simulink model "real"  (R2023a)
settings: Solver=ode1  StartTime=0.0  StopTime=inf  FixedStep=0.005  RelTol=1e-3
settings Model: SimulationMode=external  ExtModeTrigDuration=200000  Creator=5420  LastModifiedBy=zhs20
settings SolverCC: AlgebraicLoopSolver=TrustRegion
settings DataIOCC: LimitDataPoints=on  SaveFormat=Array  SignalLoggingSaveFormat=ModelDataLogs  ReturnWorkspaceOutputs=off  SignalLoggingName=sigsOut
settings OptimizationCC: ExpressionDepthLimit=2147483647  InitFltsAndDblsToZero=on
settings DebuggingCC: SaveWithParameterizedLinksMsg=none  UnderspecifiedInitializationDetection=Classic  MergeDetectMultiDrivingBlocksExec=none  SignalResolutionControl=TryResolveAllWithWarning  MultiTaskDSMMsg=warning  MultiTaskCondExecSysMsg=none  UnconnectedInputMsg=warning  UnconnectedOutputMsg=warning  UnconnectedLineMsg=warning  StateNameClashWarn=warning  SFUnexpectedBacktrackingDiag=warning  SFNoUnconditionalDefaultTransitionDiag=warning  SFExecutionAtInitializationDiag=none  ArithmeticOperatorsInVariantConditions=warning
settings HardwareCC: ProdBitPerLong=64  ProdHWDeviceType=Intel->x86-64 (Linux 64)
settings ModelReferenceCC: PropagateSignalLabelsOutOfModel=off
settings SFSimCC: SimUseLocalCustomCode=off  CustomCodeUndefinedFunction=UseInterfaceOnly
settings RTWCC: Description=Simulink Desktop Real-Time  SystemTargetFile=sldrt.tlc  TemplateMakefile=sldrt.tmf  RTWUseLocalCustomCode=off  RTWCompilerOptimization=on
settings CodeAppCC: MaxIdLength=95  StateflowObjectComments=on
settings SimulinkDesktopRealTimeCC: TargetLibSuffix=_sldrt.a  TargetPreCompLibLocation=C:\Program Files\MATLAB\R2023a\toolbox\sldrt\lib\win64  TargetLangStandard=C89/C90 (ANSI)  ModelReferenceCompliant=off  CompOptLevelCompliant=off  SupportVariableSizeSignals=off
settings ConfigComp: CovMetricSettings=dw  CovSaveCumulativeToWorkspaceVar=on  CovSaveSingleToWorkspaceVar=on  CovExternalEMLEnable=off

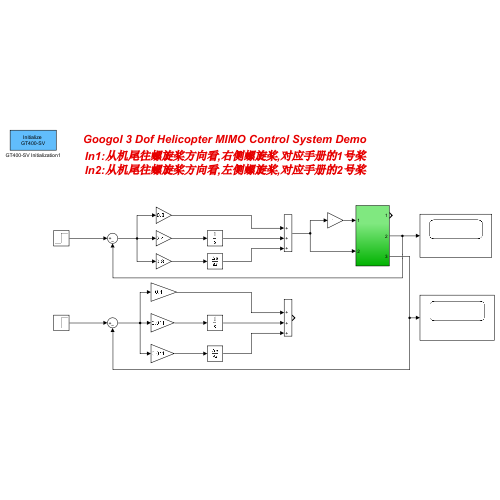
[thumbnail: Simulink's stored preview of the top-level diagram]
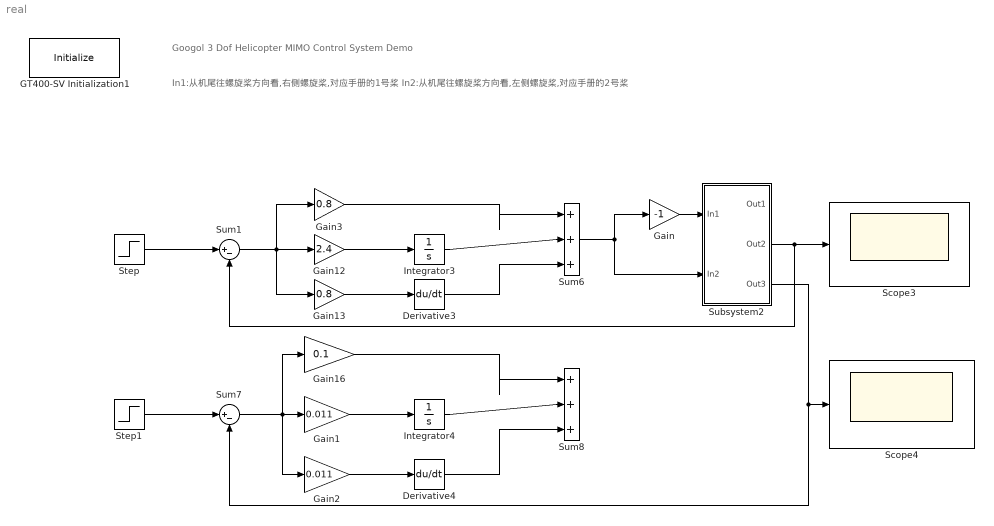
== system real ==
  note: Googol 3 Dof Helicopter MIMO Control System Demo
  note: In1:从机尾往螺旋桨方向看,右侧螺旋桨,对应手册的1号桨
      | In2:从机尾往螺旋桨方向看,左侧螺旋桨,对应手册的2号桨
  Derivative3 : Derivative
  Derivative4 : Derivative
  GT400-SV Initialization1 : S-Function  Priority=0  FunctionName=Initialize  Parameters=openloop  SFunctionDeploymentMode=off  EnableBusSupport=off  mask(Initialize){openloop=1}
      mask prompts: openloop "Control loop:"
      mask help:
      | Initializing the googol GT400-SV motion control board.
      | Block parameter:
      |     Control loop:
      |          0: closed-loop control.
      |          1: opened-loop control.
      mask Help: This initialize block initializes the googol GT400-SV motion control board.
      mask Display: disp('Initialize \nGT400-SV');
  Gain : Gain  Gain=-1
  Gain1 : Gain  Gain=0.011
  Gain12 : Gain  Gain=2.4
  Gain13 : Gain  Gain=0.8
  Gain16 : Gain  Gain=0.1
  Gain2 : Gain  Gain=0.011
  Gain3 : Gain  Gain=0.8
  Integrator3 : Integrator
  Integrator4 : Integrator
  Scope3 : Scope
  Scope4 : Scope
  Step : Step  After=0.3  SampleTime=0
  Step1 : Step  After=3  SampleTime=0
  Subsystem2 : Subsystem
  Sum1 : Sum  Inputs=|+-
  Sum6 : Sum  Inputs=|+++
  Sum7 : Sum  Inputs=|+-
  Sum8 : Sum  Inputs=|+++
  wires:
  Sum1/1 -> Gain3/1, Gain12/1, Gain13/1
  Gain12/1 -> Integrator3/1
  Gain13/1 -> Derivative3/1
  Gain3/1 -> Sum6/1
  Integrator3/1 -> Sum6/2
  Derivative3/1 -> Sum6/3
  Subsystem2/2(Out2) -> Scope3/1, Sum1/2
  Step1/1 -> Sum7/1
  Sum7/1 -> Gain2/1, Gain1/1, Gain16/1
  Gain1/1 -> Integrator4/1
  Gain2/1 -> Derivative4/1
  Gain16/1 -> Sum8/1
  Integrator4/1 -> Sum8/2
  Derivative4/1 -> Sum8/3
  Sum6/1 -> Gain/1, Subsystem2/2(In2)
  Gain/1 -> Subsystem2/1(In1)
  Subsystem2/3(Out3) -> Sum7/2, Scope4/1
  Step/1 -> Sum1/1

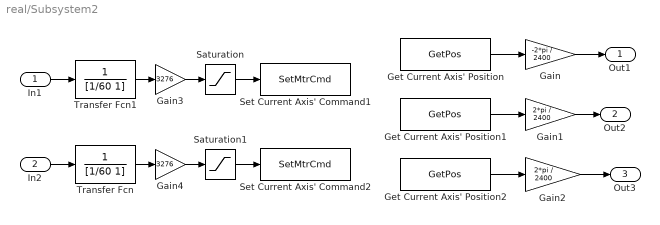
== system real/Subsystem2 ==
  In1 : Inport
  In2 : Inport  Port=2
  Gain : Gain  Gain=-2*pi / 2400  SaturateOnIntegerOverflow=on  OutDataTypeStr=Inherit: Same as input  ParamDataTypeStr=Inherit: Same as input
  Gain1 : Gain  Gain=2*pi / 2400  SaturateOnIntegerOverflow=on  OutDataTypeStr=Inherit: Same as input  ParamDataTypeStr=Inherit: Same as input
  Gain2 : Gain  Gain=2*pi / 2400  SaturateOnIntegerOverflow=on  OutDataTypeStr=Inherit: Same as input  ParamDataTypeStr=Inherit: Same as input
  Gain3 : Gain  Gain=3276
  Gain4 : Gain  Gain=3276
  Get Current Axis' Position : S-Function  Priority=1  FunctionName=GetPos  Parameters=axis  SFunctionDeploymentMode=off  EnableBusSupport=off  mask(GetPos){axis=2}
      mask prompts: axis "Axis number:"
      mask help:
      | Getting the current axis position value in encoder' counts.
      | Block parameter:
      |     Axis number:  must be between 1 and 6, default is 1.
      | Block output:
      |     1~4: current axis' encoder reading counts.
      |     5/6: assistant encoder 1/2 reading counts.
      mask Help:
      | This block, GetPos, is intended for getting the current axis position value in encoder' counts. This value represents the actual position for the axis
      | at the current sample time. This command operates for all profile modes.
      | The value returned is a 32-bit signed number with units of counts.
      | The range is -1,073,741,824 to 1,073,741,823.
      | 
      | You can recalculate obtained value into meter units via multiplication by the scaler coefficient .
      | 
      | Block parameter:
      |     Axis number:  must be between 1 and 4, default is 1.
      | Block input: none.
      | Block output:
      |         1~4: current axis' encoder reading counts.
      |         5/6: assistant encoder 1/2 reading counts.
      mask Display:
      | disp('GetPos');
      | port_label('output', 1, 'Pos');
  Get Current Axis' Position1 : S-Function  Priority=1  FunctionName=GetPos  Parameters=axis  SFunctionDeploymentMode=off  EnableBusSupport=off  mask(GetPos){axis=1}
      mask prompts: axis "Axis number:"
      mask help:
      | Getting the current axis position value in encoder' counts.
      | Block parameter:
      |     Axis number:  must be between 1 and 6, default is 1.
      | Block output:
      |     1~4: current axis' encoder reading counts.
      |     5/6: assistant encoder 1/2 reading counts.
      mask Help:
      | This block, GetPos, is intended for getting the current axis position value in encoder' counts. This value represents the actual position for the axis
      | at the current sample time. This command operates for all profile modes.
      | The value returned is a 32-bit signed number with units of counts.
      | The range is -1,073,741,824 to 1,073,741,823.
      | 
      | You can recalculate obtained value into meter units via multiplication by the scaler coefficient .
      | 
      | Block parameter:
      |     Axis number:  must be between 1 and 4, default is 1.
      | Block input: none.
      | Block output:
      |         1~4: current axis' encoder reading counts.
      |         5/6: assistant encoder 1/2 reading counts.
      mask Display:
      | disp('GetPos');
      | port_label('output', 1, 'Pos');
  Get Current Axis' Position2 : S-Function  Priority=1  FunctionName=GetPos  Parameters=axis  SFunctionDeploymentMode=off  EnableBusSupport=off  mask(GetPos){axis=3}
      mask prompts: axis "Axis number:"
      mask help:
      | Getting the current axis position value in encoder' counts.
      | Block parameter:
      |     Axis number:  must be between 1 and 6, default is 1.
      | Block output:
      |     1~4: current axis' encoder reading counts.
      |     5/6: assistant encoder 1/2 reading counts.
      mask Help:
      | This block, GetPos, is intended for getting the current axis position value in encoder' counts. This value represents the actual position for the axis
      | at the current sample time. This command operates for all profile modes.
      | The value returned is a 32-bit signed number with units of counts.
      | The range is -1,073,741,824 to 1,073,741,823.
      | 
      | You can recalculate obtained value into meter units via multiplication by the scaler coefficient .
      | 
      | Block parameter:
      |     Axis number:  must be between 1 and 4, default is 1.
      | Block input: none.
      | Block output:
      |         1~4: current axis' encoder reading counts.
      |         5/6: assistant encoder 1/2 reading counts.
      mask Display:
      | disp('GetPos');
      | port_label('output', 1, 'Pos');
  Saturation : Saturate  UpperLimit=9000  LowerLimit=0
  Saturation1 : Saturate  UpperLimit=9000  LowerLimit=0
  Set Current Axis' Command1 : S-Function  Priority=1  FunctionName=SetMtrCmd  Parameters=axis  SFunctionDeploymentMode=off  EnableBusSupport=off  mask(SetMtrCmd){axis=1}
      mask prompts: axis "Axis number:"
      mask help:
      | Settting the current axis' voltage.
      | Block parameter:
      |     Axis number:  must be between 1 and 4, default is 1.
      | Block input:
      |     the current axis' voltage.
      mask Help:
      | This SetMtrCmd settting the current axis' voltage.
      | Block parameter:
      |     Axis number:  must be between 1 and 4, default is 1.
      mask Display:
      | disp('          SetMtrCmd');
      | port_label('input', 1, 'Vol');
  Set Current Axis' Command2 : S-Function  Priority=1  FunctionName=SetMtrCmd  Parameters=axis  SFunctionDeploymentMode=off  EnableBusSupport=off  mask(SetMtrCmd){axis=2}
      mask prompts: axis "Axis number:"
      mask help:
      | Settting the current axis' voltage.
      | Block parameter:
      |     Axis number:  must be between 1 and 4, default is 1.
      | Block input:
      |     the current axis' voltage.
      mask Help:
      | This SetMtrCmd settting the current axis' voltage.
      | Block parameter:
      |     Axis number:  must be between 1 and 4, default is 1.
      mask Display:
      | disp('          SetMtrCmd');
      | port_label('input', 1, 'Vol');
  Transfer Fcn : TransferFcn  Denominator=[1/60 1]
  Transfer Fcn1 : TransferFcn  Denominator=[1/60 1]
  Out1 : Outport
  Out2 : Outport  Port=2
  Out3 : Outport  Port=3
  wires:
  Transfer Fcn1/1 -> Gain3/1
  Transfer Fcn/1 -> Gain4/1
  Saturation1/1 -> Set Current Axis' Command2/1
  Gain4/1 -> Saturation1/1
  Saturation/1 -> Set Current Axis' Command1/1
  Gain3/1 -> Saturation/1
  In1/1 -> Transfer Fcn1/1
  In2/1 -> Transfer Fcn/1
  Gain2/1 -> Out3/1
  Gain1/1 -> Out2/1
  Gain/1 -> Out1/1
  Get Current Axis' Position2/1 -> Gain2/1
  Get Current Axis' Position1/1 -> Gain1/1
  Get Current Axis' Position/1 -> Gain/1
